simulink model "DVS"  (Simulink 7.3)
settings: Solver=ode45  StartTime=0.0  StopTime=10.0  RelTol=1e-3
settings Model: Creator=Sainquake Notebook  LastModifiedBy=Sainquake Notebook

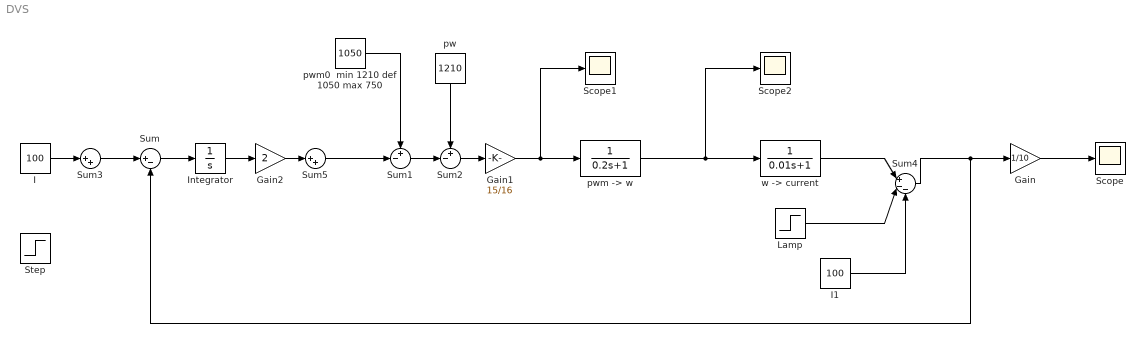
== system DVS ==
  Gain : Gain  Gain=1/10  ParameterDataType=fixdt(1, 16)  ParameterScaling=2^0  OutDataType=fixdt(1, 16)  OutScaling=2^0
  Gain1 : Gain  Gain=15/16  ParameterDataType=fixdt(1, 16)  ParameterScaling=2^0  OutDataType=fixdt(1, 16)  OutScaling=2^0
  Gain2 : Gain  Gain=2  ParameterDataType=fixdt(1, 16)  ParameterScaling=2^0  OutDataType=fixdt(1, 16)  OutScaling=2^0
  I : Constant  Value=100  OutDataType=fixdt(1, 16)  OutScaling=2^0
  I1 : Constant  Value=100  OutDataType=fixdt(1, 16)  OutScaling=2^0
  Integrator : Integrator
  Lamp : Step  Time=5  After=100  SampleTime=0
  Scope : Scope
  Scope1 : Scope
  Scope2 : Scope
      settings: SaveName=ScopeData2
  Step : Step  Time=5  After=100  SampleTime=0
  Sum : Sum  Inputs=|+-  OutDataType=fixdt(1, 16)  OutScaling=2^0
  Sum1 : Sum  Inputs=+-|  OutDataType=fixdt(1, 16)  OutScaling=2^0
  Sum2 : Sum  Inputs=+-|  OutDataType=fixdt(1, 16)  OutScaling=2^0
  Sum3 : Sum  Inputs=|++  OutDataType=fixdt(1, 16)  OutScaling=2^0
  Sum4 : Sum  Inputs=|+--  OutDataType=fixdt(1, 16)  OutScaling=2^0
  Sum5 : Sum  Inputs=|++  OutDataType=fixdt(1, 16)  OutScaling=2^0
  "pw " : Constant  Value=1210  OutDataType=fixdt(1, 16)  OutScaling=2^0
  "pwm -> w" : TransferFcn  Denominator=[0.2 1]
  pwm0  min 1210 def 1050 max 750 : Constant  Value=1050  OutDataType=fixdt(1, 16)  OutScaling=2^0
  "w -> current" : TransferFcn  Denominator=[0.01 1]
  wires:
  "pwm -> w"/1 -> "w -> current"/1, Scope2/1
  Sum/1 -> Integrator/1
  pwm0  min 1210 def 1050 max 750/1 -> Sum1/1
  Gain/1 -> Scope/1
  Sum2/1 -> Gain1/1
  Sum1/1 -> Sum2/2
  "pw "/1 -> Sum2/1
  Gain1/1 -> "pwm -> w"/1, Scope1/1
  Sum3/1 -> Sum/1
  Gain2/1 -> Sum5/1
  Sum5/1 -> Sum1/2
  Integrator/1 -> Gain2/1
  I/1 -> Sum3/1
  "w -> current"/1 -> Sum4/1
  Sum4/1 -> Gain/1, Sum/2
  Lamp/1 -> Sum4/2
  I1/1 -> Sum4/3
